simulink model "v01velocitySourceHarmonicDrive"  (R2016b)
settings: Solver=VariableStepAuto  StartTime=0.0  StopTime=10.0  RelTol=1e-3  AbsTol=1e-3  EnableMultiTasking=on
libraries: fl_lib x7, nesl_utility x4, sdl_lib x1
settings Model: Creator=Taeke  LastModifiedBy=Taeke
settings DataIOCC: LimitDataPoints=on
settings OptimizationCC: LifeSpan=inf
settings DebuggingCC: AllowSymbolicDim=off  SFUnexpectedBacktrackingDiag=warning  SFNoUnconditionalDefaultTransitionDiag=warning  SFExecutionAtInitializationDiag=none
settings GRTTargetCC: TargetLangStandard=C89/C90 (ANSI)  GeneratePreprocessorConditionals=Disable all
settings ConfigComp: CovMetricSettings=dw  CovHtmlReporting=on  CovSaveCumulativeToWorkspaceVar=on  CovSaveSingleToWorkspaceVar=on  CovExternalEMLEnable=off  CovSFcnEnable=off
settings SimscapeCC: SimscapeLogType=all  SimscapeLogDataHistory=10000

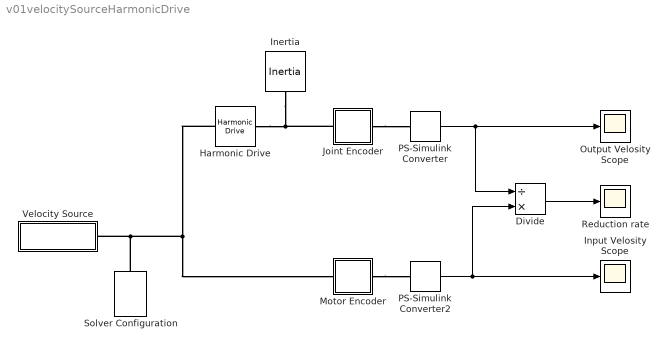
== system v01velocitySourceHarmonicDrive ==
  Divide : Product  Inputs=/*
  Harmonic Drive : sdl_lib/Gears/Harmonic Drive  n_ellipse=100  n_circle=101  friction_model=2  T_noload=0.1 N*m  T_nom=5 N*m  efficiency_nom=.95  efficiency=.95  mu_visc=[0.1, 0.1] N*m/(rad/s)  w_thr=0.01 rad/s  pwr_thr=0.001 W  temperature_TLU=[280.0, 300.0, 320.0] K  load_TLU=[1.0, 5.0, 10.0] N*m  efficiency_TLU=[0.95, 0.9, 0.85]  efficiency_TLU2=[0.85, 0.8, 0.75; 0.95, 0.9, 0.85; 0.85, 0.8, 0.7]  thermal_mass=50 J/K  T_init=300 K
  Inertia : fl_lib/Mechanical/Rotational Elements/Inertia  inertia=5 kg*m^2  w_specify=on  w_priority=Low  w=0 rad/s  t_specify=off  t_priority=None  t=0 N*m
  Input Velosity Scope : Scope
  Joint Encoder : Subsystem
  Motor Encoder : Subsystem
  Output Velosity Scope : Scope
  PS-Simulink Converter : nesl_utility/PS-Simulink Converter  PhysicalDomain=network_engine_domain  SubClassName=ps_output  LeftPortType=input  RightPortType=output  PseudoPeriodic=off  Frequencies=[]  Unit=1  AffineConversion=off
  PS-Simulink Converter2 : nesl_utility/PS-Simulink Converter  PhysicalDomain=network_engine_domain  SubClassName=ps_output  LeftPortType=input  RightPortType=output  PseudoPeriodic=off  Frequencies=[]  Unit=1  AffineConversion=off
  Reduction rate : Scope
  Solver Configuration : nesl_utility/Solver Configuration  PhysicalDomain=network_engine_domain  SubClassName=solver  LeftPortType=input  RightPortType=generic  Accelerate=off  Tones=[]  Harmonics=[]  SimulateNoise=off  Profile=off  UseLocalSampling=off  EnableSwitchedLinearOptims=on  FrequencyDomain=off  UseCCode=off  RelTol=0.001  AbsTol=1e-06  MinStep=1e-09  ToWorkspace=off  RevertToSquareIcSolve=off  NumHomotopyIterations=100  PhasorMode=off  PhasorModeNumHarmonics=1  OverrideAbsTol=off  DoDC=off  ResidualTolerance=1e-09  UseLocalSolver=off  LocalSolverChoice=NE_BACKWARD_EULER_ADVANCER  LocalSolverSampleTime=0.001  DoFixedCost=off  MaxNonlinIter=3  MaxModeIter=2  LinearAlgebra=Sparse  DelaysMemoryBudget=1024  AutomaticFiltering=on  FilteringTimeConstant=0.001
  Velocity Source : Subsystem  mask(Rotation Velocity Source){inputVelocity=100}
      mask prompts: inputVelocity "Constant Velosity [rad/s]"
      mask help: A source which generate a constant rotational velocity.
      mask init:
      | initialVelocity = 0;
  wires:
  PS-Simulink Converter/1 -> Output Velosity Scope/1, Divide/1
  Divide/1 -> Reduction rate/1
  PS-Simulink Converter2/1 -> Divide/2, Input Velosity Scope/1
  connections:
  Joint Encoder/LConn1 -- Harmonic Drive/RConn1 -- Inertia/LConn1
  Joint Encoder/RConn1 -- PS-Simulink Converter/LConn1
  Motor Encoder/RConn1 -- PS-Simulink Converter2/LConn1
  Harmonic Drive/LConn1 -- Velocity Source/LConn1 -- Solver Configuration/RConn1 -- Motor Encoder/LConn1

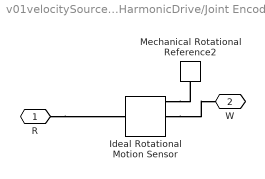
== system v01velocitySourceHarmonicDrive/Joint Encoder ==
  Ideal Rotational Motion Sensor : fl_lib/Mechanical/Mechanical Sensors/Ideal Rotational Motion Sensor  offset=0 rad
  Mechanical Rotational Reference2 : fl_lib/Mechanical/Rotational Elements/Mechanical Rotational Reference
  R : PMIOPort  Port=1  Side=Left
  W : PMIOPort  Port=2  Side=Right
  connections:
  R/RConn1 -- Ideal Rotational Motion Sensor/LConn1
  Ideal Rotational Motion Sensor/RConn1 -- Mechanical Rotational Reference2/LConn1
  Ideal Rotational Motion Sensor/RConn2 -- W/RConn1

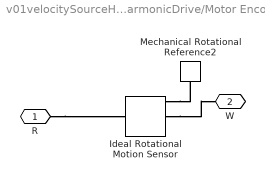
== system v01velocitySourceHarmonicDrive/Motor Encoder ==
  Ideal Rotational Motion Sensor : fl_lib/Mechanical/Mechanical Sensors/Ideal Rotational Motion Sensor  offset=0 rad
  Mechanical Rotational Reference2 : fl_lib/Mechanical/Rotational Elements/Mechanical Rotational Reference
  R : PMIOPort  Port=1  Side=Left
  W : PMIOPort  Port=2  Side=Right
  connections:
  R/RConn1 -- Ideal Rotational Motion Sensor/LConn1
  Ideal Rotational Motion Sensor/RConn1 -- Mechanical Rotational Reference2/LConn1
  Ideal Rotational Motion Sensor/RConn2 -- W/RConn1

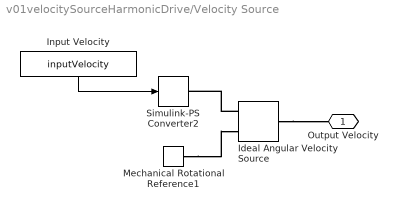
== system v01velocitySourceHarmonicDrive/Velocity Source ==
  Ideal Angular Velocity Source : fl_lib/Mechanical/Mechanical Sources/Ideal Angular Velocity Source
  Input Velocity : Constant  Value=inputVelocity
  Mechanical Rotational Reference1 : fl_lib/Mechanical/Rotational Elements/Mechanical Rotational Reference
  Simulink-PS Converter2 : nesl_utility/Simulink-PS Converter  PhysicalDomain=network_engine_domain  SubClassName=ps_input  LeftPortType=input  RightPortType=output  PseudoPeriodic=off  Frequencies=[]  NoiseDistribution=none  NoiseParameters=[]  Unit=1  AffineConversion=off  InputFiltering=off  SimscapeFilterOrder=1  InputFilterTimeConstant=0.001  UdotUserProvided=1
  Output Velocity : PMIOPort  Port=1  Side=Left
  wires:
  Input Velocity/1 -> Simulink-PS Converter2/1
  connections:
  Ideal Angular Velocity Source/RConn1 -- Simulink-PS Converter2/RConn1
  Mechanical Rotational Reference1/LConn1 -- Ideal Angular Velocity Source/RConn2
  Ideal Angular Velocity Source/LConn1 -- Output Velocity/RConn1
